simulink model "linmodel_eq1"  (R2019a)
settings: Solver=VariableStepAuto  StartTime=0.0  StopTime=30  RelTol=1e-3
InitFcn:
  | lin_discr_model
values from neighbouring files (symbols this model uses):
  A_eq1 = [0 0 1 0 ... (first row only)    [lin_discr_model.m]
  A_eq1_d = real(A_eq1_d)    [lin_discr_model.m]
  B = [0 0 ... (first row only)    [lin_discr_model.m]
  B_eq1_d = real(B_eq1_d)    [lin_discr_model.m]
  C = [1 0 0 0 ... (first row only)    [lin_discr_model.m]
  C_d = C    [lin_discr_model.m]
undefined symbols (not defined in the file or in its folder): Continuous, Time
libraries: ctrlSharedLib x1
settings Model: Creator=jessi  LastModifiedBy=jessi

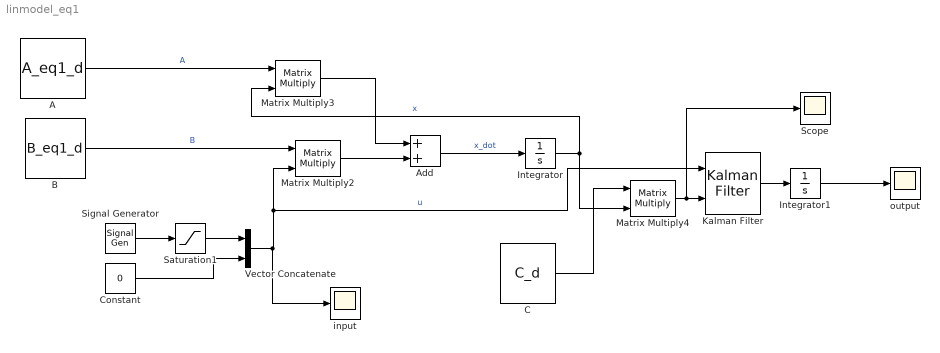
== system linmodel_eq1 ==
  A : Constant  Value=A_eq1_d
  Add : Sum
  B : Constant  Value=B_eq1_d
  C : Constant  Value=C_d
  Constant : Constant  Value=0
  Integrator : Integrator  InitialCondition=[pi;0;0;0]
  Integrator1 : Integrator
  Kalman Filter : ctrlSharedLib/Kalman Filter  TimeDomain=Continuous-Time  UseCurrentEstimator=on  ModelSource=Individual A, B, C, D matrices  ModelSourceVariable=ss(0.95,1,1,0,1)  A=A_eq1  B=B  C=C  D=0  NumberOfStates=1  NumberOfInputs=1  NumberOfOutputs=1  InitialEstimateSource=Dialog  X0=[pi;0;0;0]  P0=10  UseK=off  UseGH=off  NumberOfProcessNoiseInputs=1  G=1  TimeInvariantG=on  H=0  TimeInvariantH=on  Q=0.05  TimeInvariantQ=on  R=1  TimeInvariantR=on  N=0  TimeInvariantN=on  AddInputPort=on  AddEnablePort=off  OutputEstimatedY=off  OutputP=off  Ts=-1
      settings: SourceProductBaseCode=CT
  Matrix Multiply2 : Product  Multiplication=Matrix(*)
  Matrix Multiply3 : Product  Multiplication=Matrix(*)
  Matrix Multiply4 : Product  Multiplication=Matrix(*)
  Saturation1 : Saturate  UpperLimit=1  LowerLimit=-1
  Scope : Scope
  Signal Generator : SignalGenerator  WaveForm=square  Amplitude=0.3
  Vector Concatenate : Concatenate
  input : Scope
  output : Scope
  wires:
  B/1 -> Matrix Multiply2/1  "B"
  Matrix Multiply2/1 -> Add/2
  A/1 -> Matrix Multiply3/1  "A"
  Add/1 -> Integrator/1  "x_dot"
  Integrator/1 -> Matrix Multiply4/2, Matrix Multiply3/2  "x"
  Matrix Multiply3/1 -> Add/1
  Constant/1 -> Vector Concatenate/2
  Vector Concatenate/1 -> input/1, Kalman Filter/1, Matrix Multiply2/2  "u"
  C/1 -> Matrix Multiply4/1
  Signal Generator/1 -> Saturation1/1
  Kalman Filter/1 -> Integrator1/1
  Integrator1/1 -> output/1
  Saturation1/1 -> Vector Concatenate/1
  Matrix Multiply4/1 -> Scope/1, Kalman Filter/2
